simulink model "lab4p2a"  (R2023b)
settings: Solver=ode23tb  StartTime=0.0  StopTime=Tmdl  FixedStep=To/100  MaxStep=To/100  RelTol=1e-3
undefined symbols (not defined in the file or in its folder): an, dsc, k, To
settings Model: Creator=deniskirbaba  LastModifiedBy=Max

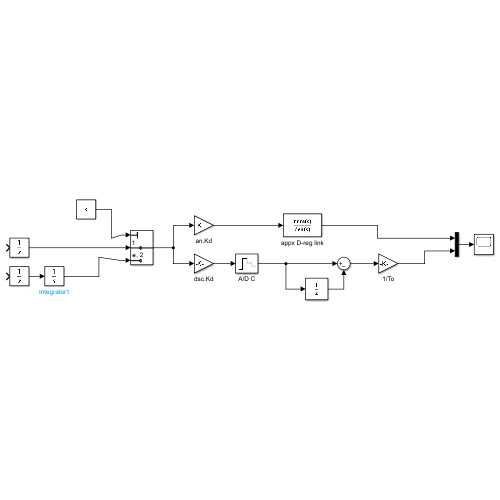
[thumbnail: Simulink's stored preview of the top-level diagram]
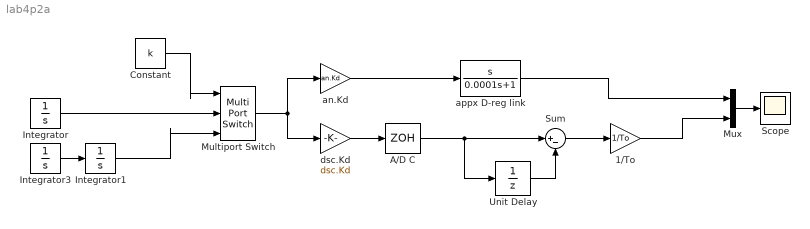
== system lab4p2a ==
  1/To : Gain  Gain=1/To
  A/D C : ZeroOrderHold  SampleTime=To
  Constant : Constant  Value=k
  Integrator : Integrator  InitialCondition=1
  Integrator1 : Integrator
  Integrator3 : Integrator  InitialCondition=1
  Multiport Switch : MultiPortSwitch  Inputs=2  SaturateOnIntegerOverflow=off  InputSameDT=off
  Mux : Mux  Inputs=2
  Scope : Scope
  Sum : Sum  Inputs=|+-
  Unit Delay : UnitDelay  SampleTime=To  HasFrameUpgradeWarning=on
  an.Kd : Gain  Gain=an.Kd
  appx D-reg link : TransferFcn  Numerator=[1 0]  Denominator=[0.0001 1]
  dsc.Kd : Gain  Gain=dsc.Kd
  wires:
  an.Kd/1 -> appx D-reg link/1
  Mux/1 -> Scope/1
  appx D-reg link/1 -> Mux/1
  Multiport Switch/1 -> dsc.Kd/1, an.Kd/1
  dsc.Kd/1 -> A/D C/1
  Unit Delay/1 -> Sum/2
  A/D C/1 -> Unit Delay/1, Sum/1
  Sum/1 -> 1/To/1
  1/To/1 -> Mux/2
  Integrator3/1 -> Integrator1/1
  Constant/1 -> Multiport Switch/1
  Integrator1/1 -> Multiport Switch/3
  Integrator/1 -> Multiport Switch/2
